simulink model "PTC_MBDS_MeanValueT_RE_Sample"  (R2013a)
settings: Solver=FixedStepDiscrete  StartTime=0.0  StopTime=100  FixedStep=Auto  RelTol=1e-3
undefined symbols (not defined in the file): sigbuilder_block
libraries: simulink_extras x1, PTC_MBDS_LIB x1
settings Model: Creator=uidl7367  LastModifiedBy=sundeep.tuteja
settings DataIOCC: SignalLoggingSaveFormat=ModelDataLogs
settings OptimizationCC: ExpressionDepthLimit=2147483647  InitFltsAndDblsToZero=on
settings DebuggingCC: SaveWithParameterizedLinksMsg=none  SignalResolutionControl=TryResolveAllWithWarning  SolverPrmCheckMsg=none  InheritedTsInSrcMsg=none  MultiTaskDSMMsg=warning  MultiTaskCondExecSysMsg=none  FcnCallInpInsideContextMsg=UseLocalSettings  StrictBusMsg=Warning
settings RTWCC: IncludeERTFirstTime=on
settings GRTTargetCC: TargetFcnLib=ansi_tfl_tmw.mat  CombineOutputUpdateFcns=off  GRTInterface=on

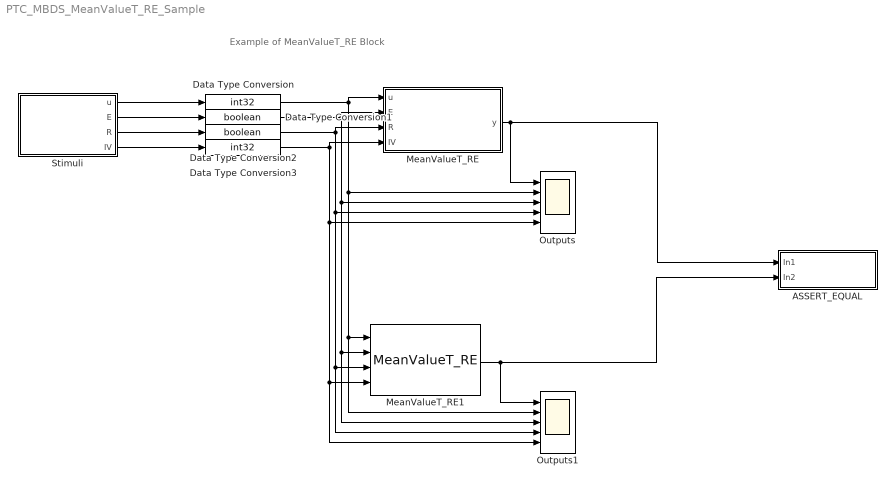
== system PTC_MBDS_MeanValueT_RE_Sample ==
  note: Example of MeanValueT_RE Block
  ASSERT_EQUAL : Subsystem
  Data Type Conversion : DataTypeConversion  InitFcn=|  OutDataTypeStr=int32  SaturateOnIntegerOverflow=on
      | try
      |    MBDS_BlockCallback('Update', gcb);
      | end
  Data Type Conversion1 : DataTypeConversion  InitFcn=|  OutDataTypeStr=boolean  SaturateOnIntegerOverflow=on
      | try
      |    MBDS_BlockCallback('Update', gcb);
      | end
  Data Type Conversion2 : DataTypeConversion  InitFcn=|  OutDataTypeStr=boolean  SaturateOnIntegerOverflow=on
      | try
      |    MBDS_BlockCallback('Update', gcb);
      | end
  Data Type Conversion3 : DataTypeConversion  InitFcn=|  OutDataTypeStr=int32  SaturateOnIntegerOverflow=on
      | try
      |    MBDS_BlockCallback('Update', gcb);
      | end
  MeanValueT_RE : Subsystem  InitFcn=|  mask(MeanValueT_RE){MBDS_LibraryBlock=on, E_Enabled=on, R_Enabled=on, IV_Enabled=on, IV=0, K=10, MBDS_BlockVersion=05.40}
      | if(exist('MBDS_BlockCallback', 'file'))
      |    MBDS_BlockCallback('Update', gcb);
      | end
      mask prompts: MBDS_LibraryBlock "MBDS library block"; E_Enabled "Show E Port"; R_Enabled "Show R Port"; IV_Enabled "Show IV Port"; IV "Initial value (IV):"; K "Average window length (K):"; MBDS_BlockVersion "Block version:"
      mask help: The output value y is the arithmetic mean value of the K most recent samples of the input signal.
      mask init:
      | if(exist('MBDS_BlockCallback', 'file'))
      |    MBDS_BlockCallback('Init', gcb);
      | else
      |    % Disable all mask parameters
      |    MaskEnables = get_param(gcb, 'MaskEnables');
      |    for k = [1:length(MaskEnables)]
      |       MaskEnables{k} = 'off';
      |    end
      |    if(~isequal(MaskEnables, get_param(gcb, 'MaskEnables')))
      |       set_param(gcb, 'MaskEnables', MaskEnables);
      |    end
      | end
      settings: AttributesFormatString=K = %<K>
      mask Help: eval(['open([workdir(''library_dir:''),''\Blockset\help\'',get_param(gcb,''MaskType''),''.html''])'])
      mask Callback R_Enabled:
      | if(exist('MBDS_BlockCallback', 'file'))
      |    MBDS_BlockCallback('R_Enabled', gcb);
      | end
      mask Callback IV_Enabled:
      | if(exist('MBDS_BlockCallback', 'file'))
      |    MBDS_BlockCallback('IV_Enabled', gcb);
      | end
      mask Callback IV:
      | % Adopt Value
      | if(exist('MBDS_BlockCallback', 'file'))
      |    MBDS_BlockCallback('IV', gcb);
      | end
      mask Callback K:
      | % Adopt Value
      | if(exist('MBDS_BlockCallback', 'file'))
      |    MBDS_BlockCallback('K', gcb);
      | end
      mask Display:
      | % Show icon or block text
      | if(exist('MeanValue.tif', 'file'))
      |    image(imread('MeanValue.tif','tif'), [0.32712215320911 0.225 0.31304347826087 0.55]);
      |    disp('')
      | else
      |    disp(sprintf('Mean\nValue'));
      | end
      | 
      | % Display port labels
      | port_label('input', 1, 'u');
      | port_label('input', 2, 'E');
      | port_label('input', 3, 'R');
      | port_label('input', 4, 'IV');
      | port_label('output', 1, 'y');
  MeanValueT_RE1 : PTC_MBDS_LIB/MBDS Standard Library/Basic Operations/Non-Linear Operations/MeanValueT_RE  E_Enabled=on  R_Enabled=on  IV_Enabled=on  IV=0  K_Enabled=off  K=10  K_prev=10  PTC_MBDS_BlockVersion=5.32  PTC_BlockType=PTC_MBDS_MeanValueT_RE
      settings: AttributesFormatString=K = %<K>
  Outputs : Scope  NumInputPorts=5
      settings: TimeRange=100  YMin=-5~-5~0~0~0  YMax=5~5~1~1~2  SampleInput=on  SampleTime=1
  Outputs1 : Scope  NumInputPorts=5
      settings: TimeRange=100  YMin=-5~-5~0~0~0  YMax=5~5~1~1~2  SampleInput=on  SampleTime=1
  Stimuli : Subsystem  Tag=STV Subsys  LoadFcn=sigbuilder_block('load');  StartFcn=sigbuilder_block('start');  StopFcn=sigbuilder_block('stop');  ClipboardFcn=sigbuilder_block('clipboard');  mask(Sigbuilder block){}
      mask help: Sigbuilder GUI
      mask init:
      | if ~strcmp(get_param(bdroot(gcb),'SimulationStatus'),'stopped') tuvar = sigbuilder_block('maskInit'); end
      settings: CopyFcn=sigbuilder_block('copy');  DeleteFcn=sigbuilder_block('delete');  ModelCloseFcn=sigbuilder_block('modelClose');  PreSaveFcn=sigbuilder_block('preSave');  PauseFcn=sigbuilder_block('pause')  ContinueFcn=sigbuilder_block('continue')  NameChangeFcn=sigbuilder_block('namechange');  OpenFcn=sigbuilder_block('open',[39 333.75 726 283.5 ]);  CloseFcn=sigbuilder_block('close');
      mask Display: plot(0,0,100,100,[10,10,40,40,10],[80,20,20,80,80],[40,10],[50,50], [40,27,10],[65,72,56],[40,25,25,10],[28,28,43,43]);
  wires:
  Data Type Conversion/1 -> MeanValueT_RE/1(u), MeanValueT_RE1/1, Outputs1/2, Outputs/2
  Data Type Conversion1/1 -> MeanValueT_RE/2(E), MeanValueT_RE1/2, Outputs1/3, Outputs/3
  Stimuli/1(u) -> Data Type Conversion/1
  Stimuli/2(E) -> Data Type Conversion1/1
  Stimuli/3(R) -> Data Type Conversion2/1
  Stimuli/4(IV) -> Data Type Conversion3/1
  Data Type Conversion2/1 -> MeanValueT_RE/3(R), Outputs1/4, MeanValueT_RE1/3, Outputs/4
  Data Type Conversion3/1 -> MeanValueT_RE/4(IV), MeanValueT_RE1/4, Outputs1/5, Outputs/5
  MeanValueT_RE/1(y) -> Outputs/1, ASSERT_EQUAL/1(In1)
  MeanValueT_RE1/1 -> ASSERT_EQUAL/2(In2), Outputs1/1

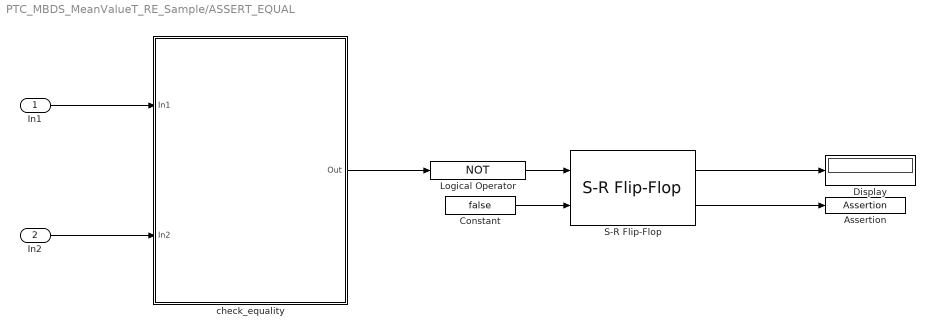
== system PTC_MBDS_MeanValueT_RE_Sample/ASSERT_EQUAL ==
  In1 : Inport
  In2 : Inport  Port=2
  Assertion : Assertion
  Constant : Constant  Value=false
  Display : Display
  Logical Operator : Logic  Operator=NOT  AllPortsSameDT=off  OutDataTypeStr=boolean
  S-R Flip-Flop : simulink_extras/Flip Flops/S-R Flip-Flop  initial_condition=0
  check_equality : MATLAB Function  TreatAsAtomicUnit=on
  wires:
  S-R Flip-Flop/1 -> Display/1
  check_equality/1(Out) -> Logical Operator/1
  Constant/1 -> S-R Flip-Flop/2
  S-R Flip-Flop/2 -> Assertion/1
  In2/1 -> check_equality/2(In2)
  In1/1 -> check_equality/1(In1)
  Logical Operator/1 -> S-R Flip-Flop/1

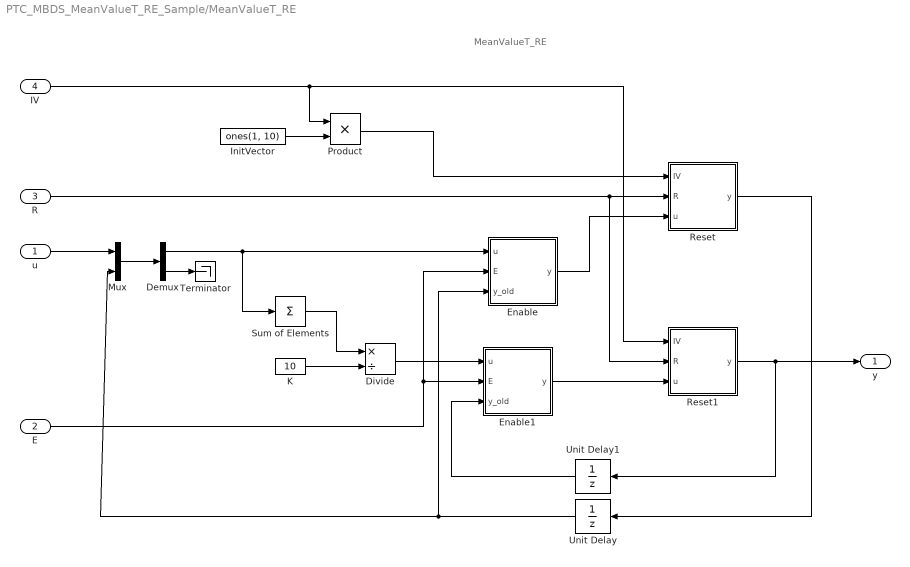
== system PTC_MBDS_MeanValueT_RE_Sample/MeanValueT_RE ==
  note: MeanValueT_RE
  u : Inport
  E : Inport  Port=2  OutDataTypeStr=boolean
  R : Inport  Port=3  OutDataTypeStr=boolean
  IV : Inport  Port=4
  Demux : Demux  Outputs=[-1 1]
  Divide : Product  Inputs=*/  OutDataTypeStr=Inherit: Inherit via back propagation
  Enable : Subsystem
  Enable1 : Subsystem
  InitVector : Constant  Value=ones(1, 10)  OutDataTypeStr=Inherit: Inherit via back propagation
  K : Constant  Value=10  OutDataTypeStr=Inherit: Inherit via back propagation
  Mux : Mux  Inputs=2
  Product : Product  OutDataTypeStr=Inherit: Inherit via back propagation
  Reset : Subsystem
  Reset1 : Subsystem
  Sum of Elements : Sum  Inputs=+  OutDataTypeStr=Inherit: Inherit via back propagation
  Terminator : Terminator
  Unit Delay : UnitDelay  SampleTime=-1
  Unit Delay1 : UnitDelay  SampleTime=-1
  y : Outport
  wires:
  E/1 -> Enable/2(E), Enable1/2(E)
  R/1 -> Reset1/2(R), Reset/2(R)
  Unit Delay1/1 -> Enable1/3(y_old)
  Reset/1(y) -> Unit Delay/1
  Product/1 -> Reset/1(IV)
  Enable/1(y) -> Reset/3(u)
  Enable1/1(y) -> Reset1/3(u)
  Divide/1 -> Enable1/1(u)
  Reset1/1(y) -> Unit Delay1/1, y/1
  K/1 -> Divide/2
  Sum of Elements/1 -> Divide/1
  InitVector/1 -> Product/2
  Demux/1 -> Sum of Elements/1, Enable/1(u)
  Demux/2 -> Terminator/1
  Mux/1 -> Demux/1
  u/1 -> Mux/1
  Unit Delay/1 -> Mux/2, Enable/3(y_old)
  IV/1 -> Product/1, Reset1/1(IV)

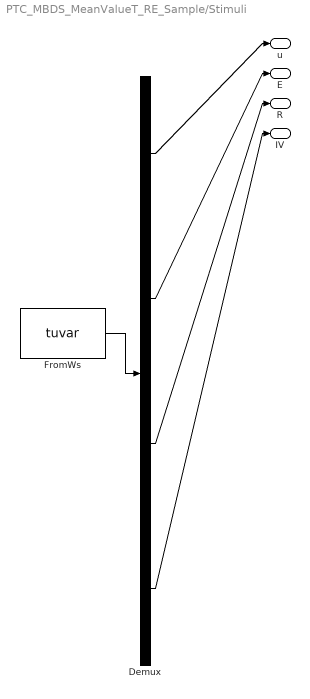
== system PTC_MBDS_MeanValueT_RE_Sample/Stimuli ==
  Demux : Demux  Tag=STV Demux
  FromWs : FromWorkspace  Tag=STV FromWs  VariableName=tuvar  SampleTime=1  OutputAfterFinalValue=Holding final value
      SigBuilderData=|
      | common.afterFinalStr = 'Hold final value'
      | common.sampleTime = 1
      | dataSet.timeRange = [0 100]
      | dataSet.name = 'test data'
      | sbobj.Groups.Name = 'test data'
      | sbobj.Groups.Signals(1).Name = 'u'
      | sbobj.Groups.Signals(1).XData = [0 5 10 15 20 25 30 35 40 45 50 55 60 65 70 75 80 85 90 95 100]
      | sbobj.Groups.Signals(1).YData = [0 2.5 3.5 3.5 2.4 0 -2.4 -3.5 -3.5 -2.4 0 2.9381016588 4.7549388855 4.75565465343 2.93997557915 0 -2.93772679904 -4.75479560945 -4.75579768454 -2.94035028752 0]
      | sbobj.Groups.Signals(2).Name = 'E'
      | sbobj.Groups.Signals(2).XData = [0 5 5 10 10 100]
      | sbobj.Groups.Signals(2).YData = [1 1 0 0 1 1]
      | sbobj.Groups.Signals(3).Name = 'R'
      | sbobj.Groups.Signals(3).XData = [0 20 20 23 23 84.8 84.8 86 86 100]
      | sbobj.Groups.Signals(3).YData = [0 0 1 1 0 0 1 1 0 0]
      | sbobj.Groups.Signals(4).Name = 'IV'
      | sbobj.Groups.Signals(4).XData = [0 64.6 64.6 100]
      | sbobj.Groups.Signals(4).YData = [0 0 2 2]
  u : Outport  Tag=STV Outport
  E : Outport  Tag=STV Outport  Port=2
  R : Outport  Tag=STV Outport  Port=3
  IV : Outport  Tag=STV Outport  Port=4
  wires:
  Demux/4 -> IV/1
  Demux/3 -> R/1
  Demux/2 -> E/1
  Demux/1 -> u/1
  FromWs/1 -> Demux/1

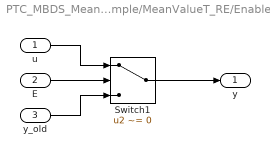
== system PTC_MBDS_MeanValueT_RE_Sample/MeanValueT_RE/Enable ==
  u : Inport
  E : Inport  Port=2
  y_old : Inport  Port=3
  Switch1 : Switch  Criteria=u2 ~= 0  OutDataTypeStr=Inherit: Inherit via back propagation  InputSameDT=on
  y : Outport
  wires:
  y_old/1 -> Switch1/3
  Switch1/1 -> y/1
  u/1 -> Switch1/1
  E/1 -> Switch1/2

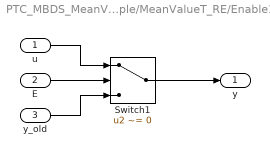
== system PTC_MBDS_MeanValueT_RE_Sample/MeanValueT_RE/Enable1 ==
  u : Inport
  E : Inport  Port=2
  y_old : Inport  Port=3
  Switch1 : Switch  Criteria=u2 ~= 0  OutDataTypeStr=Inherit: Inherit via back propagation  InputSameDT=on
  y : Outport
  wires:
  y_old/1 -> Switch1/3
  Switch1/1 -> y/1
  u/1 -> Switch1/1
  E/1 -> Switch1/2

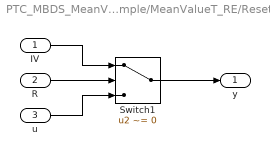
== system PTC_MBDS_MeanValueT_RE_Sample/MeanValueT_RE/Reset ==
  IV : Inport
  R : Inport  Port=2
  u : Inport  Port=3
  Switch1 : Switch  Criteria=u2 ~= 0  OutDataTypeStr=Inherit: Inherit via back propagation  InputSameDT=on
  y : Outport
  wires:
  u/1 -> Switch1/3
  Switch1/1 -> y/1
  IV/1 -> Switch1/1
  R/1 -> Switch1/2

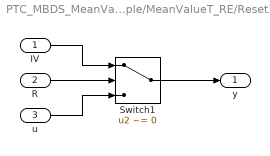
== system PTC_MBDS_MeanValueT_RE_Sample/MeanValueT_RE/Reset1 ==
  IV : Inport
  R : Inport  Port=2
  u : Inport  Port=3
  Switch1 : Switch  Criteria=u2 ~= 0  OutDataTypeStr=Inherit: Inherit via back propagation  InputSameDT=on
  y : Outport
  wires:
  u/1 -> Switch1/3
  Switch1/1 -> y/1
  IV/1 -> Switch1/1
  R/1 -> Switch1/2

== matlab function PTC_MBDS_MeanValueT_RE_Sample/ASSERT_EQUAL/check_equality ==
  data: In1 input; Out output; In2 input
function Out = check_equality(In1, In2)
%#codegen

Out = isequaln(In1, In2);

end
